simulink model "DC_PID"  (R2022b)
settings: Solver=FixedStepAuto  StartTime=0.0  StopTime=t_max  FixedStep=timestep  RelTol=1e-3
values from neighbouring files (symbols this model uses):
  den = [J*La (Ra*J+B*La) (Ra*B+Kb^2) 0]    [DC_MOTOR_analisys.m]
  K = double(solve(A,k))    [DC_MOTOR_analisys.m]
  num = Kb    (= 1.2)    [DC_MOTOR_analisys.m]
  step_v = 1    [DC_MOTOR_analisys.m]
undefined symbols (not defined in the file or in its folder): Kp, Td, Ti
settings Model: Creator=mluser  LastModifiedBy=mluser
settings SolverCC: AlgebraicLoopSolver=TrustRegion
settings DebuggingCC: ArithmeticOperatorsInVariantConditions=warning
settings SFSimCC: CustomCodeUndefinedFunction=UseInterfaceOnly
settings CodeAppCC: StateflowObjectComments=on

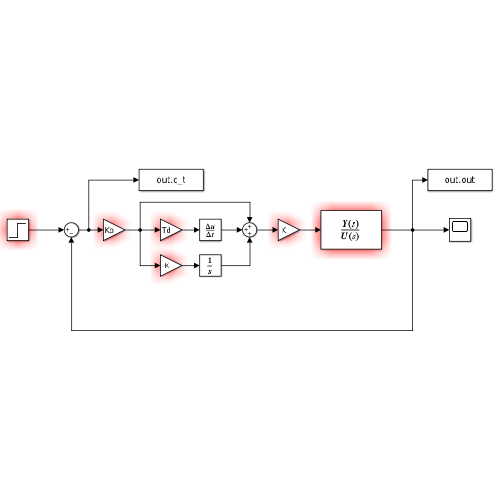
[thumbnail: Simulink's stored preview of the top-level diagram]
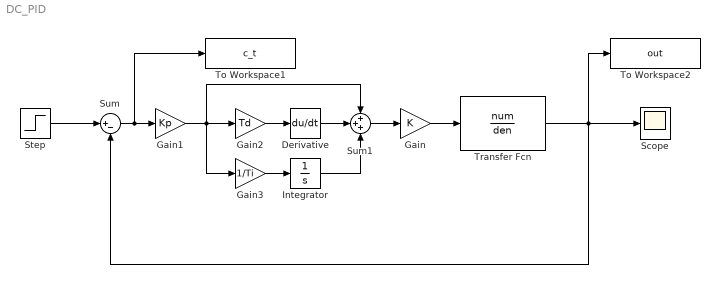
== system DC_PID ==
  Derivative : Derivative
  Gain : Gain  Gain=K
  Gain1 : Gain  Gain=Kp
  Gain2 : Gain  Gain=Td
  Gain3 : Gain  Gain=1/Ti
  Integrator : Integrator
  Scope : Scope
  Step : Step  Time=0  After=step_v  SampleTime=0
  Sum : Sum  Inputs=|+-
  Sum1 : Sum  Inputs=+++
  To Workspace1 : ToWorkspace  VariableName=c_t  SampleTime=-1
  To Workspace2 : ToWorkspace  VariableName=out  SampleTime=-1
  Transfer Fcn : TransferFcn  Numerator=num  Denominator=den
  wires:
  Transfer Fcn/1 -> Scope/1, To Workspace2/1, Sum/2
  Step/1 -> Sum/1
  Gain/1 -> Transfer Fcn/1
  Sum1/1 -> Gain/1
  Sum/1 -> Gain1/1, To Workspace1/1
  Gain1/1 -> Gain3/1, Sum1/1, Gain2/1
  Gain2/1 -> Derivative/1
  Derivative/1 -> Sum1/2
  Gain3/1 -> Integrator/1
  Integrator/1 -> Sum1/3
